simulink model "SC_I"  (R2021b)
settings: Solver=VariableStepAuto  StartTime=0.0  StopTime=10.0  RelTol=1e-3
values from neighbouring files (symbols this model uses):
  d = [5.5 1 0.05]    [I_matrix_data.m]    (also in a.m)
  MB = [50 1 1 1]    [I_matrix_data.m]    (also in a.m)
  SP = [10 10 1 0.1 0]    [I_matrix_data.m]    (also in a.m)
settings Model: Creator=adity  LastModifiedBy=adity

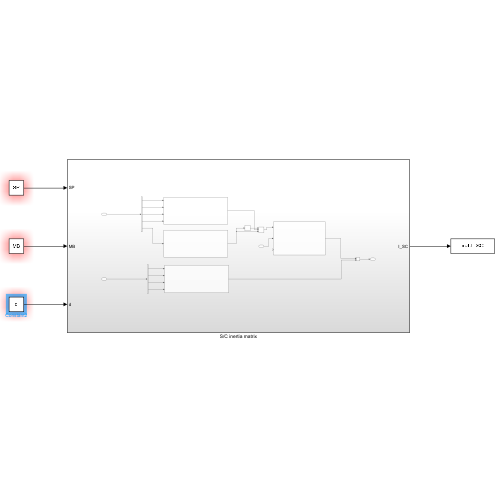
[thumbnail: Simulink's stored preview of the top-level diagram]
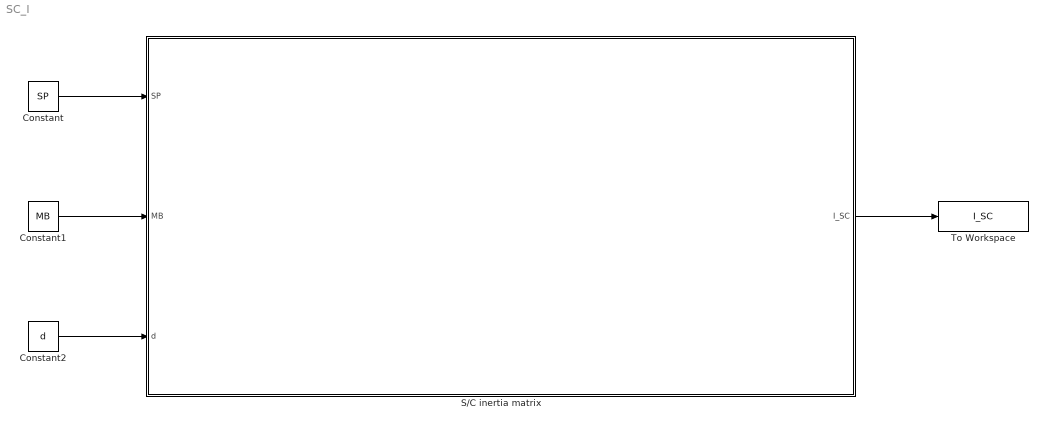
== system SC_I ==
  Constant : Constant  Value=SP
  Constant1 : Constant  Value=MB
  Constant2 : Constant  Value=d
  S/C inertia matrix : Subsystem
  To Workspace : ToWorkspace  VariableName=I_SC  SaveFormat=Timeseries  SampleTime=-1
  wires:
  Constant2/1 -> S/C inertia matrix/3(d)
  Constant1/1 -> S/C inertia matrix/2(MB)
  S/C inertia matrix/1(I_SC) -> To Workspace/1
  Constant/1 -> S/C inertia matrix/1(SP)

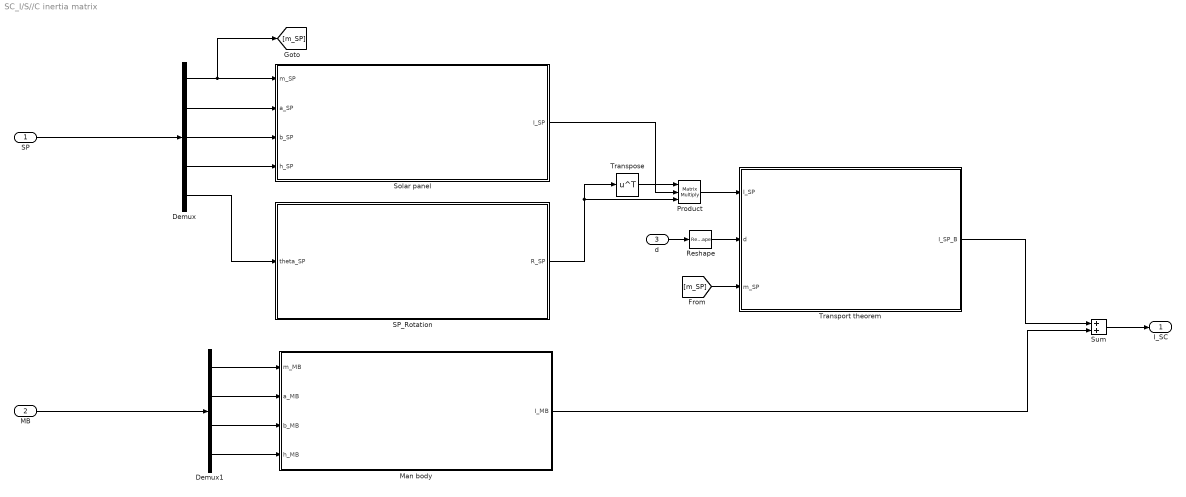
== system SC_I/S//C inertia matrix ==
  SP : Inport
  MB : Inport  Port=2
  d : Inport  Port=3
  Demux : Demux  Outputs=5
  Demux1 : Demux
  Man body : Subsystem
  Product : Product  Inputs=3  Multiplication=Matrix(*)
  Reshape : Reshape  OutputDimensionality=Column vector (2-D)
  SP_Rotation : Subsystem
  Solar panel : Subsystem
  Sum : Sum
  Transport theorem : Subsystem
  Transpose : Math  Operator=transpose  SaturateOnIntegerOverflow=on
  I_SC : Outport
  wires:
  SP_Rotation/1(R_SP) -> Transpose/1, Product/3
  Solar panel/1(I_SP) -> Product/2
  Transpose/1 -> Product/1
  Demux/1 -> [m_SP], Solar panel/1(m_SP)
  Demux/2 -> Solar panel/2(a_SP)
  Demux/3 -> Solar panel/3(b_SP)
  Demux/4 -> Solar panel/4(h_SP)
  SP/1 -> Demux/1
  Demux/5 -> SP_Rotation/1(theta_SP)
  Demux1/1 -> Man body/1(m_MB)
  Demux1/2 -> Man body/2(a_MB)
  Demux1/3 -> Man body/3(b_MB)
  Demux1/4 -> Man body/4(h_MB)
  MB/1 -> Demux1/1
  Product/1 -> Transport theorem/1(I_SP)
  d/1 -> Reshape/1
  Sum/1 -> I_SC/1
  Transport theorem/1(I_SP_B) -> Sum/1
  Man body/1(I_MB) -> Sum/2
  Reshape/1 -> Transport theorem/2(d)
  [m_SP] -> Transport theorem/3(m_SP)

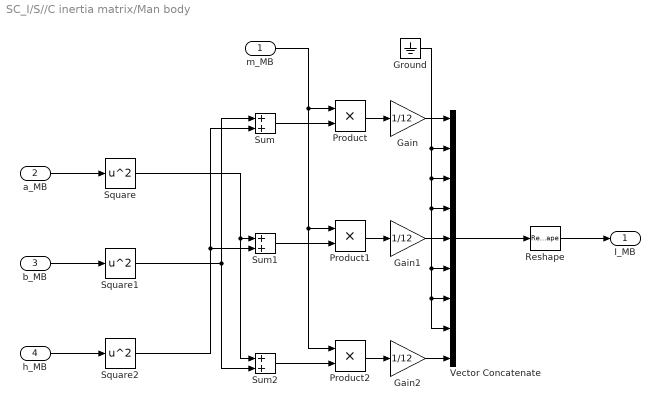
== system SC_I/S//C inertia matrix/Man body ==
  m_MB : Inport
  a_MB : Inport  Port=2
  b_MB : Inport  Port=3
  h_MB : Inport  Port=4
  Gain : Gain  Gain=1/12
  Gain1 : Gain  Gain=1/12
  Gain2 : Gain  Gain=1/12
  Ground : Ground
  Product : Product
  Product1 : Product
  Product2 : Product
  Reshape : Reshape  OutputDimensionality=Customize  OutputDimensions=[3,3]
  Square : Math  Operator=square  SaturateOnIntegerOverflow=on
  Square1 : Math  Operator=square  SaturateOnIntegerOverflow=on
  Square2 : Math  Operator=square  SaturateOnIntegerOverflow=on
  Sum : Sum
  Sum1 : Sum
  Sum2 : Sum
  Vector Concatenate : Concatenate  NumInputs=9
  I_MB : Outport
  wires:
  Ground/1 -> Vector Concatenate/2, Vector Concatenate/3, Vector Concatenate/7, Vector Concatenate/8, Vector Concatenate/6, Vector Concatenate/4
  Square/1 -> Sum2/1, Sum1/1
  Square1/1 -> Sum2/2, Sum/1
  Square2/1 -> Sum/2, Sum1/2
  Product1/1 -> Gain1/1
  Gain/1 -> Vector Concatenate/1
  Product2/1 -> Gain2/1
  Sum1/1 -> Product1/2
  m_MB/1 -> Product/1, Product2/1, Product1/1
  Sum2/1 -> Product2/2
  a_MB/1 -> Square/1
  Vector Concatenate/1 -> Reshape/1
  Sum/1 -> Product/2
  b_MB/1 -> Square1/1
  Gain1/1 -> Vector Concatenate/5
  Product/1 -> Gain/1
  Gain2/1 -> Vector Concatenate/9
  Reshape/1 -> I_MB/1
  h_MB/1 -> Square2/1

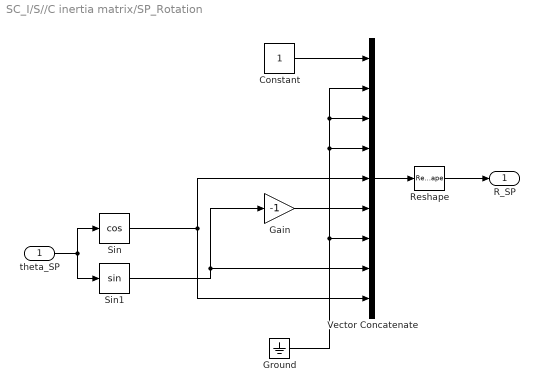
== system SC_I/S//C inertia matrix/SP_Rotation ==
  theta_SP : Inport
  Constant : Constant
  Gain : Gain  Gain=-1
  Ground : Ground
  Reshape : Reshape  OutputDimensionality=Customize  OutputDimensions=[3,3]
  Sin : Trigonometry  Operator=cos
  Sin1 : Trigonometry
  Vector Concatenate : Concatenate  NumInputs=9
  R_SP : Outport
  wires:
  Vector Concatenate/1 -> Reshape/1
  Reshape/1 -> R_SP/1
  Constant/1 -> Vector Concatenate/1
  Ground/1 -> Vector Concatenate/7, Vector Concatenate/4, Vector Concatenate/3, Vector Concatenate/2
  theta_SP/1 -> Sin1/1, Sin/1
  Gain/1 -> Vector Concatenate/6
  Sin/1 -> Vector Concatenate/5, Vector Concatenate/9
  Sin1/1 -> Gain/1, Vector Concatenate/8

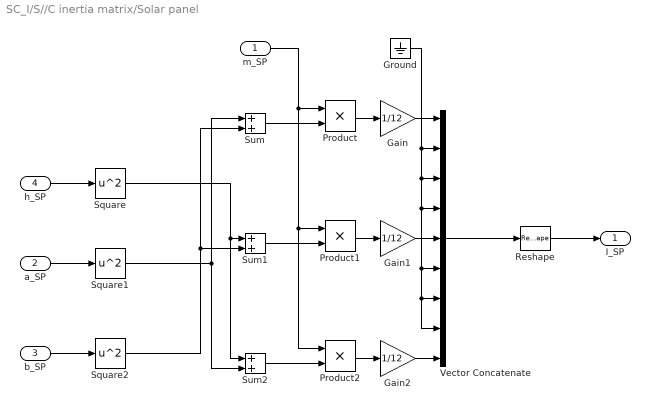
== system SC_I/S//C inertia matrix/Solar panel ==
  m_SP : Inport
  a_SP : Inport  Port=2
  b_SP : Inport  Port=3
  h_SP : Inport  Port=4
  Gain : Gain  Gain=1/12
  Gain1 : Gain  Gain=1/12
  Gain2 : Gain  Gain=1/12
  Ground : Ground
  Product : Product
  Product1 : Product
  Product2 : Product
  Reshape : Reshape  OutputDimensionality=Customize  OutputDimensions=[3,3]
  Square : Math  Operator=square  SaturateOnIntegerOverflow=on
  Square1 : Math  Operator=square  SaturateOnIntegerOverflow=on
  Square2 : Math  Operator=square  SaturateOnIntegerOverflow=on
  Sum : Sum
  Sum1 : Sum
  Sum2 : Sum
  Vector Concatenate : Concatenate  NumInputs=9
  I_SP : Outport
  wires:
  Reshape/1 -> I_SP/1
  Vector Concatenate/1 -> Reshape/1
  m_SP/1 -> Product/1, Product2/1, Product1/1
  Product/1 -> Gain/1
  Gain/1 -> Vector Concatenate/1
  Product1/1 -> Gain1/1
  Product2/1 -> Gain2/1
  Gain2/1 -> Vector Concatenate/9
  h_SP/1 -> Square/1
  a_SP/1 -> Square1/1
  b_SP/1 -> Square2/1
  Sum/1 -> Product/2
  Sum1/1 -> Product1/2
  Sum2/1 -> Product2/2
  Ground/1 -> Vector Concatenate/2, Vector Concatenate/3, Vector Concatenate/7, Vector Concatenate/8, Vector Concatenate/6, Vector Concatenate/4
  Gain1/1 -> Vector Concatenate/5
  Square1/1 -> Sum2/2, Sum/1
  Square2/1 -> Sum/2, Sum1/2
  Square/1 -> Sum2/1, Sum1/1

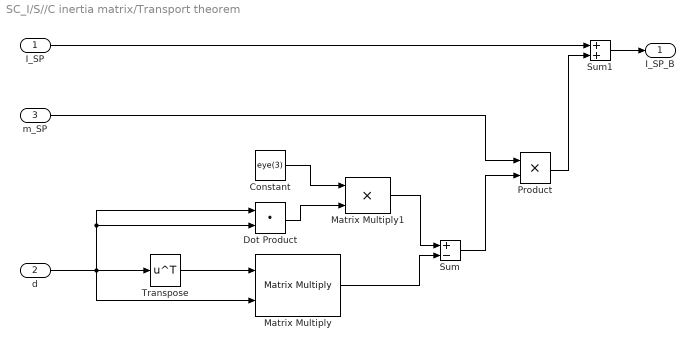
== system SC_I/S//C inertia matrix/Transport theorem ==
  I_SP : Inport
  d : Inport  Port=2
  m_SP : Inport  Port=3
  Constant : Constant  Value=eye(3)
  Dot Product : DotProduct  InputSameDT=on  OutDataTypeStr=Inherit: Inherit via internal rule
  Matrix Multiply : Product  Multiplication=Matrix(*)
  Matrix Multiply1 : Product
  Product : Product
  Sum : Sum  Inputs=+-
  Sum1 : Sum
  Transpose : Math  Operator=transpose  SaturateOnIntegerOverflow=on
  I_SP_B : Outport
  wires:
  d/1 -> Transpose/1, Dot Product/2, Dot Product/1, Matrix Multiply/2
  Transpose/1 -> Matrix Multiply/1
  Constant/1 -> Matrix Multiply1/1
  Matrix Multiply1/1 -> Sum/1
  Matrix Multiply/1 -> Sum/2
  Sum/1 -> Product/2
  m_SP/1 -> Product/1
  Product/1 -> Sum1/2
  I_SP/1 -> Sum1/1
  Sum1/1 -> I_SP_B/1
  Dot Product/1 -> Matrix Multiply1/2
